simulink model "Regenerative Braking System"  (R2019a)
settings: Solver=VariableStepDiscrete  StartTime=0.0  StopTime=10.0  RelTol=1e-3
undefined symbols (not defined in the file): c
libraries: powerlib x15, simulink x8
settings Model: Creator=USER  LastModifiedBy=USER

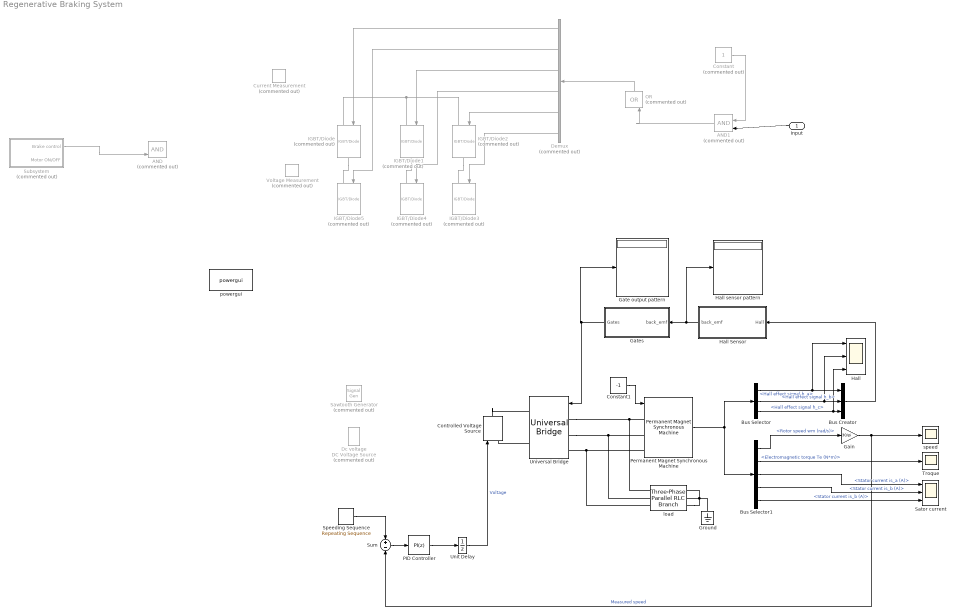
== system Regenerative Braking System ==
  Input : Inport
  " load" : powerlib/Elements/Three-Phase Parallel RLC Branch  LConnTagsString=A|B|C  RConnTagsString=A|B|C  BranchType=R  Resistance=200  Inductance=1e-3  Capacitance=1e-6  Measurements=None
      settings: SourceProductName=Simscape Electrical  SourceProductBaseCode=PS
  AND : Logic  Commented=on  IconShape=distinctive  AllPortsSameDT=off  OutDataTypeStr=boolean
  AND1 : Logic  Commented=on  IconShape=distinctive  AllPortsSameDT=off  OutDataTypeStr=boolean
  Bus Creator : BusCreator  Inputs=3
  Bus Selector : BusSelector  OutputSignals=Hall effect signal h_a,Hall effect signal h_b,Hall effect signal h_c
  Bus Selector1 : BusSelector  OutputSignals=Rotor speed wm (rad/s),Electromagnetic torque Te (N*m),Stator current is_a (A),Stator current is_b (A),Stator current is_b (A)
  Constant : Constant  Commented=on
  Constant1 : Constant  Value=-1
  Controlled Voltage Source : powerlib/Electrical Sources/Controlled Voltage Source  Initialize=on  Source_Type=AC  Amplitude=0  Phase=0  Frequency=0  Measurements=None
      settings: SourceProductName=Simscape Electrical
  Current Measurement : powerlib/Measurements/Current Measurement  Commented=on  PhasorSimulation=off  OutputType=Complex  PSBequivalent=0
      settings: SourceProductName=Simscape Electrical
  Dc voltage : powerlib/Electrical Sources/DC Voltage Source  Commented=on  Amplitude=300  Measurements=None
      settings: SourceProductName=Simscape Electrical
  Demux : Demux  Commented=on  Outputs=6
  Gain : Gain  Gain=30/pi
  Gate output pattern : Display
  Gates : Subsystem
  Ground : powerlib/Elements/Ground  LConnTagsString=a
      settings: SourceProductName=Simscape Electrical
  Hall : Scope  NumInputPorts=3
  Hall Sensor : Subsystem
  Hall sensor pattern : Display
  IGBT/Diode{,1..5} (6 alike) : powerlib/Power Electronics/IGBT//Diode  Commented=on  Ron=1e-3  Rs=1e5  Cs=inf  Measurements=off
      settings: SourceProductName=Simscape Electrical
  OR : Logic  Commented=on  Operator=OR  IconShape=distinctive  AllPortsSameDT=off  OutDataTypeStr=boolean
  PID Controller : simulink/Continuous/PID Controller  Controller=PI  Form=Parallel  TimeDomain=Discrete-time  SampleTime=-1  IntegratorMethod=Forward Euler  FilterMethod=Forward Euler  ControllerParametersSource=internal  P=0.01  I=5  D=0  UseFilter=on  N=100  TunerSelectOption=Transfer Function Based (PID Tuner App)  InitialConditionSource=internal  InitialConditionForIntegrator=0  InitialConditionForFilter=0  DifferentiatorICPrevScaledInput=0  ExternalReset=none  TrackingMode=off  Kt=1  LimitOutput=off  UpperSaturationLimit=inf  LowerSaturationLimit=-inf  LinearizeAsGain=on  AntiWindupMode=none  Kb=1  POutMin=[]  POutMax=[]  IOutMin=[]  IOutMax=[]  DOutMin=[]  DOutMax=[]  NOutMin=[]  NOutMax=[]  SumOutMin=[]  SumOutMax=[]  SaturationOutMin=[]  SaturationOutMax=[]  PParamMin=[]  PParamMax=[]  IParamMin=[]  IParamMax=[]  DParamMin=[]  DParamMax=[]  NParamMin=[]  NParamMax=[]  KbParamMin=[]  KbParamMax=[]  KtParamMin=[]  KtParamMax=[]  KbOutMin=[]  KbOutMax=[]  KtOutMin=[]  KtOutMax=[]  IntegratorOutMin=[]  IntegratorOutMax=[]  FilterOutMin=[]  FilterOutMax=[]  SumI1OutMin=[]  SumI1OutMax=[]  SumI2OutMin=[]  SumI2OutMax=[]  SumI3OutMin=[]  SumI3OutMax=[]  SumI4OutMin=[]  SumI4OutMax=[]  SumDOutMin=[]  SumDOutMax=[]  DifferentiatorOutMin=[]  DifferentiatorOutMax=[]  FilterDiffOutCoefMin=[]  FilterDiffOutCoefMax=[]  ReciprocalOutMin=[]  ReciprocalOutMax=[]  SumDenOutMin=[]  SumDenOutMax=[]  SumNumOutMin=[]  SumNumOutMax=[]  DivideOutMin=[]  DivideOutMax=[]  IntegratorContinuousStateAttributes=''  IntegratorStateMustResolveToSignalObject=off  IntegratorRTWStateStorageClass=Auto  FilterContinuousStateAttributes=''  FilterStateMustResolveToSignalObject=off  FilterRTWStateStorageClass=Auto  ParallelPVariant=InternalParameters  IdealPVariant=Disabled  IVariant=InternalParameters  DVariant=Disabled  IntegratorVariant=Discrete  SatVariant=Disabled  AWVariant=Passthrough  PCopyVariant=Disabled  TRVariant=Disabled  FdbkBlocksVariant=Forward  IdealPFdbkVariant=Disabled  SatFdbkVariant=Disabled  DerivativeFilterVariant=Disabled  NVariant=Disabled  NCopyVariant=Disabled_SignalSpec  FilterICVariant=Disabled  IntegratorICVariant=InternalICs  ExternalResetVariant=Disabled  TRSumVariant=Passthrough  SumFdbkVariant=Disabled  SumVariant=Sum_PI
  Permanent Magnet Synchronous Machine : powerlib/Machines/Permanent Magnet Synchronous Machine  NbPhases=3  FluxDistribution=Trapezoidal  RotorType=Round  MechanicalLoad=Torque Tm  PresetModel=No  ShowDetailedParameters=on  MeasurementBus=off  Resistance=2.8750  Inductance=8.5e-3  dqInductances=[8.5e-3,8.5e-3]  La=0.000395  MachineConstant=Flux linkage established by magnets (V.s)  Flux=0.175  VoltageCst=146.6077  TorqueCst=1.4  Flat=120  Mechanical=[0.8e-3 1e-3 4]  PolePairs=4  InitialConditions=[0,0, 0,0]  InitialConditions5ph=[0 0 0 0 0 0]  TsPowergui=0  TsBlock=-1  RefAngle=90 degrees behind phase A axis (modified Park)
  Sator current : Scope  NumInputPorts=3
  Sawtooth Generator : SignalGenerator  Commented=on  WaveForm=sawtooth  Units=rad/sec
  Speeding Sequence : simulink/Sources/Repeating Sequence  rep_seq_t=[0 0.5 1 1.5 2 2.5 3 3.5]  rep_seq_y=[0 1 100 300 600 700 800 900]
  Subsystem : Subsystem  Commented=on
  Sum : Sum  Inputs=+-
  Troque : Scope
  Unit Delay : UnitDelay  SampleTime=-1  HasFrameUpgradeWarning=on
  Universal Bridge : powerlib/Power Electronics/Universal Bridge  Arms=3  SnubberResistance=5000  SnubberCapacitance=1e-6  Device=MOSFET / Diodes  Ron=1e-3  Lon=0  ForwardVoltages="[  0  0  ]"  ForwardVoltage=0  GTOparameters=[ 10e-6 , 20e-6 ]  IGBTparameters=[ 1e-6 , 2e-6 ]  Measurements=None  Measurements_2=None  converterType=Rectifier
      settings: SourceProductName=Simscape Electrical
  Voltage Measurement : powerlib/Measurements/Voltage Measurement  Commented=on  PhasorSimulation=off  OutputType=Complex  PSBequivalent=0
      settings: SourceProductName=Simscape Electrical
  powergui : powerlib/powergui  Priority=1  SimulationMode=Discrete  SampleTime=50e-6  frequency=60  Iterations=50  frequencyindice=0  Pbase=100e6  ErrMax=1e-4  UnitsV=kV  UnitsW=MW  buscounter=0  FunctionMessages=off  echomessages=off  EnableUseOfTLC=off  CurrentSourceSwitches=off  DisableSnubberDevices=off  DisableRonSwitches=off  DisableVfSwitches=off  DisplayEquations=off  AutomaticDiscreteSolvers=off  SolverType=Tustin/Backward Euler (TBE)  Interpol=off  ExternalGateDelay=off  methode=off  Ts=100  x0status=blocks  SPID=on  SwTol=0  HookPort=off  NonlinearTolerance=0  nMaxIteration=15  ContinueOnMaxIteration=off  RestoreLinks=warning  ResistiveCurrentMeasurement=off  Frange=[0:2:500]  Ylog=off  Xlog=on  ShowGrid=off  save=off  variable=ZData  structure=0  ZoomFFT=off  StartTime=0.0  cycles=1  DisplayStyle=1  fundamental=60  FreqAxis=off  MaxFrequency=1000  frequencyindicesteady=1  RmsSteady=1  display=off
      settings: SourceProductName=Simscape Electrical
  speed : Scope
  wires:
  Hall Sensor/1(back_emf) -> Hall sensor pattern/1, Gates/1(back_emf)
  Gates/1(Gates) -> Gate output pattern/1, Universal Bridge/1
  Subsystem/1(Brake control) -> AND/2
  Demux/2 -> IGBT/Diode5/1
  Demux/4 -> IGBT/Diode4/1
  Demux/6 -> IGBT/Diode3/1
  Demux/5 -> IGBT/Diode2/1
  Demux/3 -> IGBT/Diode1/1
  Demux/1 -> IGBT/Diode/1
  OR/1 -> Demux/1
  AND1/1 -> OR/2
  Constant/1 -> AND1/1
  Input/1 -> AND1/2
  Permanent Magnet Synchronous Machine/1 -> Bus Selector/1, Bus Selector1/1
  Bus Selector/1 -> Hall/1, Bus Creator/1  "<Hall effect signal h_a>"
  Bus Selector/3 -> Hall/3, Bus Creator/3  "<Hall effect signal h_c>"
  Bus Creator/1 -> Hall Sensor/1(Hall)
  Constant1/1 -> Permanent Magnet Synchronous Machine/1
  Bus Selector1/1 -> Gain/1  "<Rotor speed wm (rad/s)>"
  Bus Selector1/2 -> Troque/1  "<Electromagnetic torque Te (N*m)>"
  Bus Selector1/3 -> Sator current/1  "<Stator current is_a (A)>"
  Bus Selector1/4 -> Sator current/2  "<Stator current is_b (A)>"
  Bus Selector1/5 -> Sator current/3  "<Stator current is_b (A)>"
  Sum/1 -> PID Controller/1
  PID Controller/1 -> Unit Delay/1
  Gain/1 -> speed/1, Sum/2  "Measured speed"
  Speeding Sequence/1 -> Sum/1
  Unit Delay/1 -> Controlled Voltage Source/1  "Voltage"
  Bus Selector/2 -> Hall/2, Bus Creator/2  "<Hall effect signal h_b>"
  connections:
  IGBT/Diode/RConn1 -- IGBT/Diode5/LConn1
  IGBT/Diode1/RConn1 -- IGBT/Diode4/LConn1
  IGBT/Diode2/RConn1 -- IGBT/Diode3/LConn1
  IGBT/Diode/LConn1 -- IGBT/Diode1/LConn1 -- IGBT/Diode2/LConn1
  Universal Bridge/LConn1 -- Permanent Magnet Synchronous Machine/LConn1 -- " load"/LConn1
  Universal Bridge/LConn2 -- " load"/LConn2 -- Permanent Magnet Synchronous Machine/LConn2
  Permanent Magnet Synchronous Machine/LConn3 -- Universal Bridge/LConn3 -- " load"/LConn3
  Controlled Voltage Source/RConn1 -- Universal Bridge/RConn1
  Universal Bridge/RConn2 -- Controlled Voltage Source/LConn1
  " load"/RConn3 -- " load"/RConn2 -- Ground/LConn1 -- " load"/RConn1

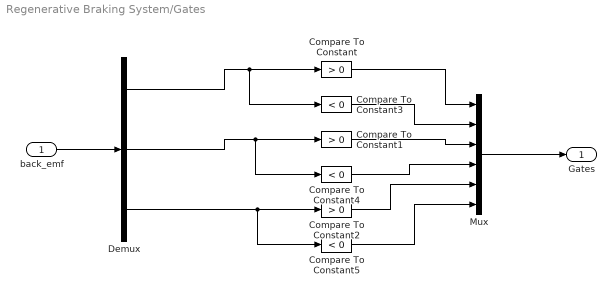
== system Regenerative Braking System/Gates ==
  back_emf : Inport
  Compare To Constant : simulink/Logic and Bit Operations/Compare To Constant  relop=>  const=0  OutDataTypeStr=boolean
  Compare To Constant1 : simulink/Logic and Bit Operations/Compare To Constant  relop=>  const=0  OutDataTypeStr=boolean
  Compare To Constant2 : simulink/Logic and Bit Operations/Compare To Constant  relop=>  const=0  OutDataTypeStr=boolean
  Compare To Constant3 : simulink/Logic and Bit Operations/Compare To Constant  relop=<  const=0  OutDataTypeStr=boolean
  Compare To Constant4 : simulink/Logic and Bit Operations/Compare To Constant  relop=<  const=0  OutDataTypeStr=boolean
  Compare To Constant5 : simulink/Logic and Bit Operations/Compare To Constant  relop=<  const=0  OutDataTypeStr=boolean
  Demux : Demux  Outputs=3
  Mux : Mux  Inputs=6
  Gates : Outport
  wires:
  Compare To Constant1/1 -> Mux/3
  Mux/1 -> Gates/1
  Compare To Constant2/1 -> Mux/5
  Compare To Constant4/1 -> Mux/4
  Compare To Constant/1 -> Mux/1
  back_emf/1 -> Demux/1
  Compare To Constant5/1 -> Mux/6
  Compare To Constant3/1 -> Mux/2
  Demux/1 -> Compare To Constant3/1, Compare To Constant/1
  Demux/2 -> Compare To Constant4/1, Compare To Constant1/1
  Demux/3 -> Compare To Constant5/1, Compare To Constant2/1

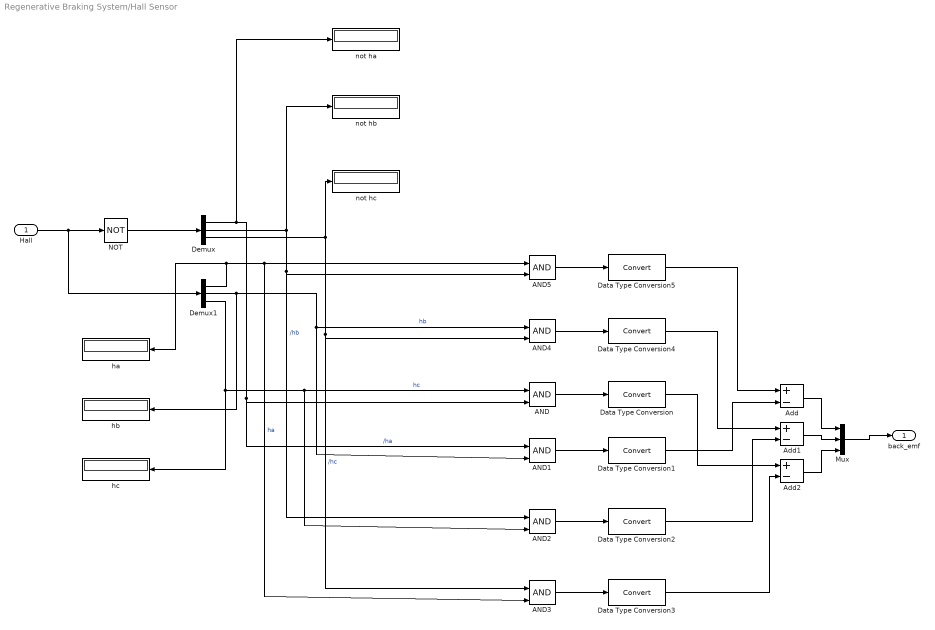
== system Regenerative Braking System/Hall Sensor ==
  Hall : Inport
  AND{,1..5} (6 alike) : Logic  IconShape=distinctive  AllPortsSameDT=off  OutDataTypeStr=boolean
  Add : Sum  Inputs=+-
  Add1 : Sum  Inputs=+-
  Add2 : Sum  Inputs=+-
  Data Type Conversion{,1..5} (6 alike) : DataTypeConversion
  Demux : Demux  Outputs=3
  Demux1 : Demux  Outputs=3
  Mux : Mux  Inputs=3
  NOT : Logic  Operator=NOT  IconShape=distinctive  AllPortsSameDT=off  OutDataTypeStr=boolean
  ha : Display
  hb : Display
  hc : Display
  not ha : Display
  not hb : Display
  not hc : Display
  back_emf : Outport
  wires:
  Demux1/1 -> ha/1, AND3/2, AND5/1  "ha"
  Data Type Conversion3/1 -> Add2/2
  Data Type Conversion5/1 -> Add/1
  AND4/1 -> Data Type Conversion4/1
  Demux1/2 -> hb/1, AND1/2, AND4/1  "hb"
  Hall/1 -> Demux1/1, NOT/1
  Demux/1 -> not ha/1, AND1/1, AND/2  "/ha"
  AND2/1 -> Data Type Conversion2/1
  Data Type Conversion/1 -> Add2/1
  AND1/1 -> Data Type Conversion1/1
  Demux1/3 -> hc/1, AND2/2, AND/1  "hc"
  Data Type Conversion4/1 -> Add1/1
  AND/1 -> Data Type Conversion/1
  NOT/1 -> Demux/1
  Data Type Conversion1/1 -> Add/2
  AND3/1 -> Data Type Conversion3/1
  Mux/1 -> back_emf/1
  Demux/3 -> AND3/1, AND4/2, not hc/1  "/hc"
  Data Type Conversion2/1 -> Add1/2
  Demux/2 -> AND5/2, AND2/1, not hb/1  "/hb"
  AND5/1 -> Data Type Conversion5/1
  Add/1 -> Mux/1
  Add1/1 -> Mux/2
  Add2/1 -> Mux/3

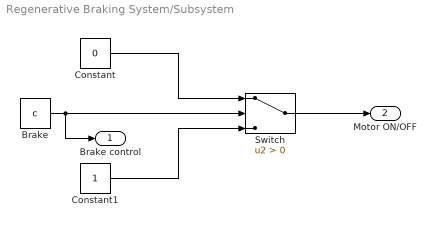
== system Regenerative Braking System/Subsystem ==
  Brake : Constant  Value=c
  Constant : Constant  Value=0
  Constant1 : Constant
  Switch : Switch  Criteria=u2 > Threshold
  Brake control : Outport
  Motor ON/OFF : Outport  Port=2
  wires:
  Brake/1 -> Brake control/1, Switch/2
  Constant/1 -> Switch/1
  Constant1/1 -> Switch/3
  Switch/1 -> Motor ON/OFF/1
